simulink model "firstCaseBlock"  (R2024b)
settings: Solver=VariableStepAuto  StartTime=0.0  StopTime=10.0  RelTol=1e-3
settings Model: Creator=ryandavis  LastModifiedBy=ryandavis

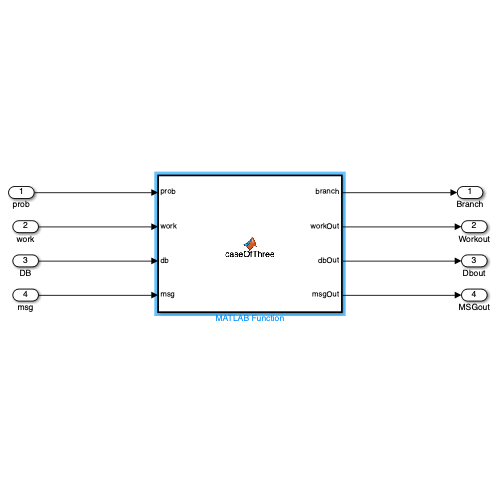
[thumbnail: Simulink's stored preview of the top-level diagram]
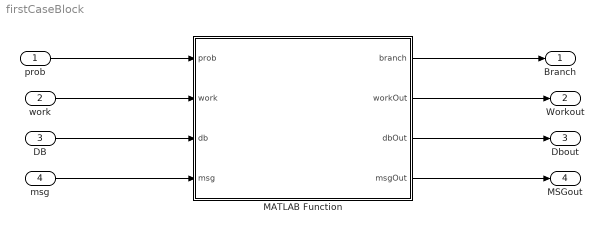
== system firstCaseBlock ==
  prob : Inport
  work : Inport  Port=2
  DB : Inport  Port=3
  msg : Inport  Port=4
  MATLAB Function : MATLAB Function  TreatAsAtomicUnit=on
  Branch : Outport
  Workout : Outport  Port=2
  Dbout : Outport  Port=3
  MSGout : Outport  Port=4
  wires:
  prob/1 -> MATLAB Function/1(prob)
  MATLAB Function/1(branch) -> Branch/1
  MATLAB Function/2(workOut) -> Workout/1
  MATLAB Function/3(dbOut) -> Dbout/1
  work/1 -> MATLAB Function/2(work)
  DB/1 -> MATLAB Function/3(db)
  msg/1 -> MATLAB Function/4(msg)
  MATLAB Function/4(msgOut) -> MSGout/1

== matlab function firstCaseBlock/MATLAB Function ==
  data: prob input; branch output; workOut output; dbOut output; work input; db input; msg input; msgOut output
function [branch, workOut, dbOut, msgOut] = caseOfThree(prob, work, db, msg)
    r = rand();

    if r < 0.5
        branch = 1; 
    elseif r < 0.9
        branch = 2;
    else
        branch = 3;
    end
    
    workOut = work;
    dbOut = db;
    msgOut = msg;
end
